simulink model "SkywalkerX8_AircraftModel_ROSGazeboAnimation"  (R2018a)
settings: Solver=FixedStepAuto  StartTime=0.0  StopTime=10  FixedStep=0.1  RelTol=1e-3
model workspace (MAT data in the model file):
  SL_ROS_VariableLengthArrays_MaxSizes.CommonInfo.ArrayTruncateAction = 'EmitWarning'
  SL_ROS_VariableLengthArrays_MaxSizes.MsgTypeMap = containers.Map
  SL_ROS_VariableLengthArrays_MaxSizes.MsgTypeMap.serialization.keys = {'gazebo_msgs/ModelState'}
  SL_ROS_VariableLengthArrays_MaxSizes.MsgTypeMap.serialization.values{1}(1).PropertyName = 'ModelName'
  SL_ROS_VariableLengthArrays_MaxSizes.MsgTypeMap.serialization.values{1}(1).DataType = 'uint8'
  SL_ROS_VariableLengthArrays_MaxSizes.MsgTypeMap.serialization.values{1}(1).MaxLength = 9
  SL_ROS_VariableLengthArrays_MaxSizes.MsgTypeMap.serialization.values{1}(2).PropertyName = 'ReferenceFrame'
  SL_ROS_VariableLengthArrays_MaxSizes.MsgTypeMap.serialization.values{1}(2).DataType = 'uint8'
  SL_ROS_VariableLengthArrays_MaxSizes.MsgTypeMap.serialization.values{1}(2).MaxLength = 128
  SL_ROS_VariableLengthArrays_MaxSizes.MsgTypeMap.serialization.uniformity = 0
  SL_ROS_VariableLengthArrays_MaxSizes.MsgTypeMap.serialization.keyType = 'char'
  SL_ROS_VariableLengthArrays_MaxSizes.MsgTypeMap.serialization.valueType = 'any'
undefined symbols (not defined in the file): ModelName, ModelName_SL_Info, Pose
libraries: robotlib x2, aerolibatmos2 x1, sharedtransform x1
settings Model: EnablePacing=on  Creator=David  LastModifiedBy=David

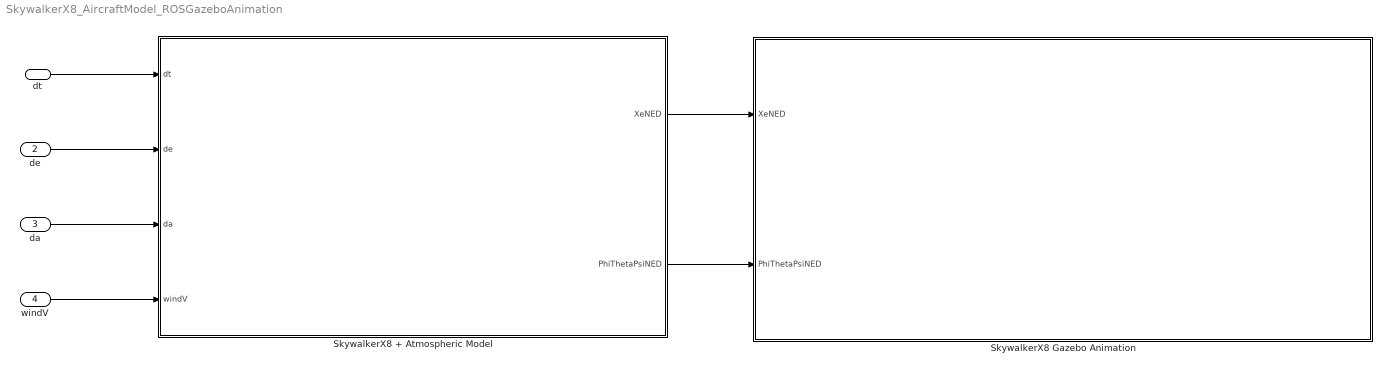
== system SkywalkerX8_AircraftModel_ROSGazeboAnimation ==
  dt : Inport
  de : Inport  Port=2
  da : Inport  Port=3
  windV : Inport  Port=4
  SkywalkerX8 + Atmospheric Model : Subsystem
      mask Display:
      | image('x8SkySunset.png', 'center')
      | 
      | port_label('input', 1, '\delta_t (Unitless)', 'texmode', 'on')
      | port_label('input', 2, '\delta_e (rad)', 'texmode', 'on')
      | port_label('input', 3, '\delta_a (rad)', 'texmode', 'on')
      | port_label('input', 4, '{\bf V_w^b} (m/s)', 'texmode', 'on')
      | 
      | port_label('output', 1, '{\bf X_e_{NED}} (m)', 'texmode', 'on')
      | port_label('output', 2, '(\phi \theta \psi)_{NED} (rad)', 'texmode', 'on')
  SkywalkerX8 Gazebo Animation : Subsystem
      mask Display:
      | image('skywalker_gazebo.png')
      | 
      | color('cyan')
      | 
      | port_label('input', 1, '{\bf X_e_{NED}} (m)', 'texmode', 'on')
      | port_label('input', 2, '(\phi \theta \psi)_{NED} (rad)', 'texmode', 'on')
  wires:
  dt/1 -> SkywalkerX8 + Atmospheric Model/1(dt)
  de/1 -> SkywalkerX8 + Atmospheric Model/2(de)
  da/1 -> SkywalkerX8 + Atmospheric Model/3(da)
  windV/1 -> SkywalkerX8 + Atmospheric Model/4(windV)
  SkywalkerX8 + Atmospheric Model/1(XeNED) -> SkywalkerX8 Gazebo Animation/1(XeNED)
  SkywalkerX8 + Atmospheric Model/2(PhiThetaPsiNED) -> SkywalkerX8 Gazebo Animation/2(PhiThetaPsiNED)

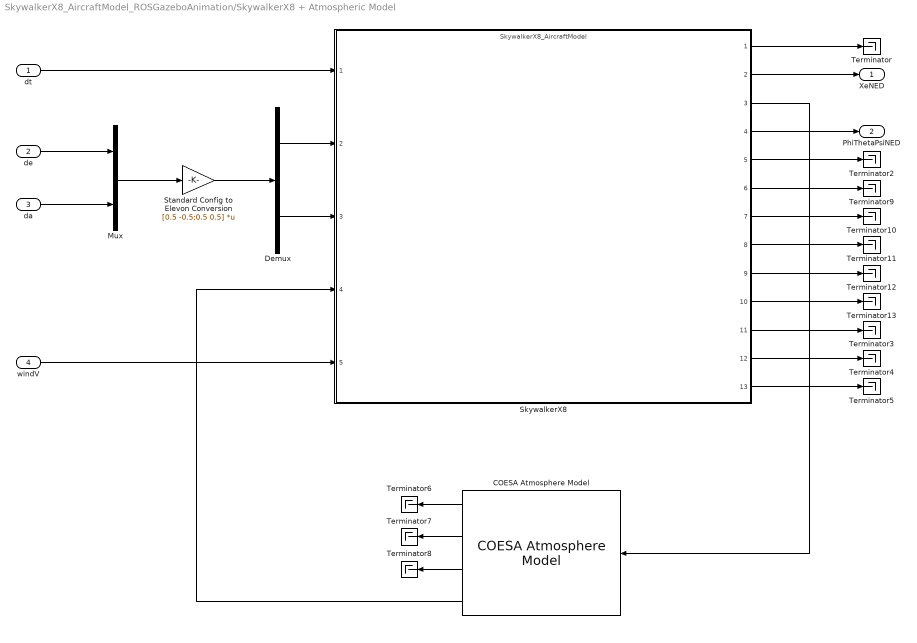
== system SkywalkerX8_AircraftModel_ROSGazeboAnimation/SkywalkerX8 + Atmospheric Model ==
  dt : Inport
  de : Inport  Port=2
  da : Inport  Port=3
  windV : Inport  Port=4
  COESA Atmosphere Model : aerolibatmos2/COESA Atmosphere Model  units=Metric (MKS)  spec=1976 COESA-extended U.S. Standard Atmosphere  model=Profile  profile_var=High temperature  profile_percent=1%  profile_alt=5 km (16404 ft)  envelope_var=High temperature  envelope_percent=1%  action=None
  Demux : Demux  Outputs=2
  Mux : Mux  Inputs=2
  SkywalkerX8 : ModelReference  ModelNameDialog=SkywalkerX8_AircraftModel  ModelReferenceVersion=1.162
      mask Display:
      | image('C:\MATLAB\masters\icons\Skywalker Main Block Icon.png', 'center')
      | 
      | color('cyan')
      | 
      | port_label('input', 1, 'k_{motor} (Unitless)', 'texmode', 'on')
      | port_label('input', 2, '\delta_{er} (rad)', 'texmode', 'on')
      | port_label('input', 3, '\delta_{el} (rad)', 'texmode', 'on')
      | port_label('input', 4, '\rho (kg/m^3)', 'texmode', 'on')
      | port_label('input', 5, '{\bf V_w^b} (m/s)', 'texmode', 'on')
      | 
      | port_label('output', 1, '{\bf V_e} (m/s)', 'texmode', 'on')
      | port_label('output', 2, '{\bf X_e} (m)', 'texmode', 'on')
      | port_label('output', 3, 'Altitude (m)', 'texmode', 'on')
      | port_label('output', 4, '\phi \theta \psi (rad)', 'texmode', 'on')
      | port_label('output', 5, 'R_{inertial}^{body}', 'texmode', 'on')
      | port_label('output', 6, 'V_a (m/s)', 'texmode', 'on')
      | port_label('output', 7, 'alpha (rad)', 'texmode', 'on')
      | port_label('output', 8, 'beta (rad)', 'texmode', 'on')
      | port_label('output', 9, '{\bf V_b} (m/s)', 'texmode', 'on')
      | port_label('output', 10, '{\bf \omega_b} (rad/s)', 'texmode', 'on')
      | port_label('output', 11, '{\bf \delta\omega_b/\deltat} (rad/s^2)', 'texmode', 'on')
      | port_label('output', 12, '{\bf a_{body}} (m/s^2)', 'texmode', 'on')
      | port_label('output', 13, '{\bf a_{inertial}} (m/s^2)', 'texmode', 'on')
  Standard Config to Elevon Conversion : Gain  Gain=[0.5 -0.5;0.5 0.5]  Multiplication=Matrix(K*u)
  Terminator{,2..13} (13 alike) : Terminator
  XeNED : Outport
  PhiThetaPsiNED : Outport  Port=2
  wires:
  SkywalkerX8/12 -> Terminator4/1
  COESA Atmosphere Model/2 -> Terminator7/1
  COESA Atmosphere Model/1 -> Terminator6/1
  Demux/2 -> SkywalkerX8/3
  SkywalkerX8/13 -> Terminator5/1
  COESA Atmosphere Model/3 -> Terminator8/1
  Mux/1 -> Standard Config to Elevon Conversion/1
  windV/1 -> SkywalkerX8/5
  SkywalkerX8/11 -> Terminator3/1
  SkywalkerX8/6 -> Terminator9/1
  COESA Atmosphere Model/4 -> SkywalkerX8/4
  SkywalkerX8/1 -> Terminator/1
  SkywalkerX8/5 -> Terminator2/1
  Standard Config to Elevon Conversion/1 -> Demux/1
  de/1 -> Mux/1
  Demux/1 -> SkywalkerX8/2
  SkywalkerX8/7 -> Terminator10/1
  dt/1 -> SkywalkerX8/1
  da/1 -> Mux/2
  SkywalkerX8/8 -> Terminator11/1
  SkywalkerX8/3 -> COESA Atmosphere Model/1
  SkywalkerX8/9 -> Terminator12/1
  SkywalkerX8/10 -> Terminator13/1
  SkywalkerX8/2 -> XeNED/1
  SkywalkerX8/4 -> PhiThetaPsiNED/1

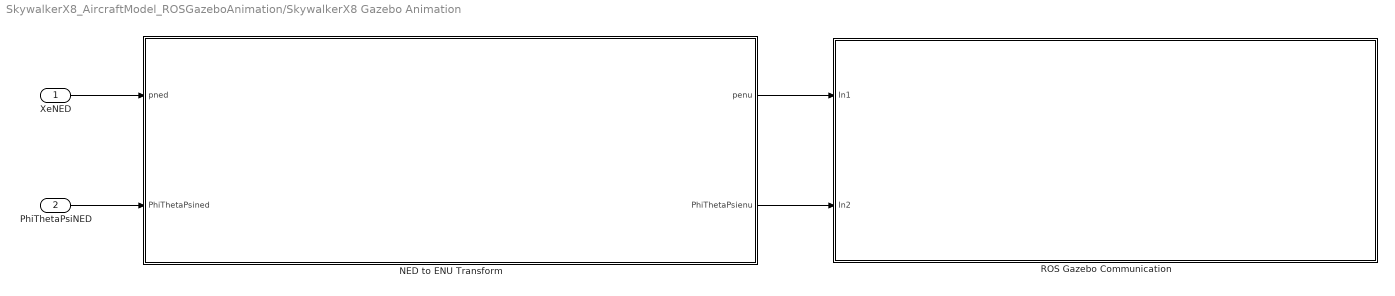
== system SkywalkerX8_AircraftModel_ROSGazeboAnimation/SkywalkerX8 Gazebo Animation ==
  XeNED : Inport
  PhiThetaPsiNED : Inport  Port=2
  "NED to ENU Transform " : Subsystem
      mask Display:
      | image('NEDtoENU.png', 'center')
      | 
      | port_label('input', 1, '{\bf X_e_{NED}} (m)', 'texmode', 'on')
      | port_label('input', 2, '(\phi \theta \psi)_{NED} (rad)', 'texmode', 'on')
      | 
      | port_label('output', 1, '{\bf X_e_{ENU}} (m)', 'texmode', 'on')
      | port_label('output', 2, '(\phi \theta \psi)_{ENU} (rad)', 'texmode', 'on')
  ROS Gazebo Communication : Subsystem
      mask Display:
      | image('rosToGazebo.png')
      | 
      | port_label('input', 1, '{\bf X_e_{ENU}} (m)', 'texmode', 'on')
      | port_label('input', 2, '(\phi \theta \psi)_{ENU} (rad)', 'texmode', 'on')
  wires:
  "NED to ENU Transform "/2(PhiThetaPsienu) -> ROS Gazebo Communication/2(In2)
  "NED to ENU Transform "/1(penu) -> ROS Gazebo Communication/1(In1)
  XeNED/1 -> "NED to ENU Transform "/1(pned)
  PhiThetaPsiNED/1 -> "NED to ENU Transform "/2(PhiThetaPsined)

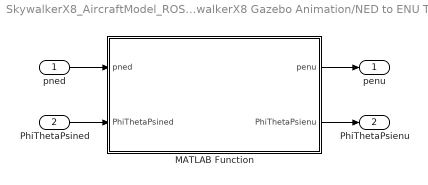
== system SkywalkerX8_AircraftModel_ROSGazeboAnimation/SkywalkerX8 Gazebo Animation/NED to ENU Transform  ==
  pned : Inport
  PhiThetaPsined : Inport  Port=2
  MATLAB Function : MATLAB Function  TreatAsAtomicUnit=on
  penu : Outport
  PhiThetaPsienu : Outport  Port=2
  wires:
  MATLAB Function/2(PhiThetaPsienu) -> PhiThetaPsienu/1
  pned/1 -> MATLAB Function/1(pned)
  MATLAB Function/1(penu) -> penu/1
  PhiThetaPsined/1 -> MATLAB Function/2(PhiThetaPsined)

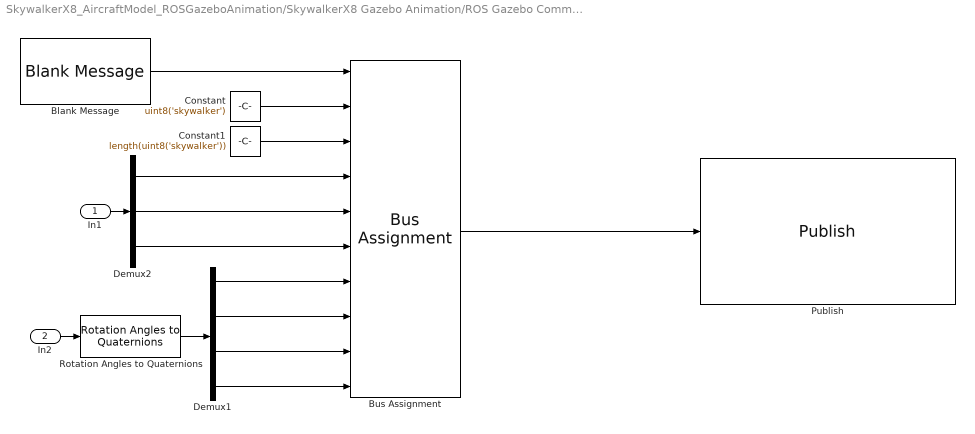
== system SkywalkerX8_AircraftModel_ROSGazeboAnimation/SkywalkerX8 Gazebo Animation/ROS Gazebo Communication ==
  In1 : Inport
  In2 : Inport  Port=2
  Blank Message : robotlib/Blank Message  SourceLibraryInfo=This block requires Robotics System Toolbox  messageType=gazebo_msgs/ModelState  SampleTime=inf
      settings: SourceProductBaseCode=RO
  Bus Assignment : BusAssignment  AssignedSignals=ModelName,ModelName_SL_Info.CurrentLength,Pose.Position.X,Pose.Position.Y,Pose.Position.Z,Pose.Orientation.W,Pose.Orientation.X,Pose.Orientation.Y,Pose.Orientation.Z
  Constant : Constant  Value=uint8('skywalker')
  Constant1 : Constant  Value=length(uint8('skywalker'))  OutDataTypeStr=uint32
  Demux1 : Demux
  Demux2 : Demux  Outputs=3
  Publish : robotlib/Publish  SourceLibraryInfo=This block requires Robotics System Toolbox  topicSource=Select from ROS network  topic=/gazebo/set_model_state  messageType=gazebo_msgs/ModelState  messageQueueLength=1
      settings: SourceProductBaseCode=RO
  Rotation Angles to Quaternions : sharedtransform/Rotation Angles to Quaternions  rotationOrder=XYZ  aMode=aMode
      settings: SourceProductName=Aerospace Blockset  SourceProductBaseCode=AE
  wires:
  Demux2/3 -> Bus Assignment/6
  Constant1/1 -> Bus Assignment/3
  Demux1/4 -> Bus Assignment/10
  Demux1/1 -> Bus Assignment/7
  In1/1 -> Demux2/1
  Demux2/1 -> Bus Assignment/4
  Demux1/2 -> Bus Assignment/8
  Bus Assignment/1 -> Publish/1
  In2/1 -> Rotation Angles to Quaternions/1
  Constant/1 -> Bus Assignment/2
  Blank Message/1 -> Bus Assignment/1
  Rotation Angles to Quaternions/1 -> Demux1/1
  Demux1/3 -> Bus Assignment/9
  Demux2/2 -> Bus Assignment/5

== matlab function SkywalkerX8_AircraftModel_ROSGazeboAnimation/SkywalkerX8 Gazebo Animation/NED to ENU Transform /MATLAB Function ==
  data: pned input size=[1, 3]; penu output size=[1, 3]; PhiThetaPsined input; PhiThetaPsienu output
function [penu, PhiThetaPsienu] = f_NEDtoENU(pned, PhiThetaPsined)

%% Description %%

% This function takes in global coordinates and rotation in the NED (North
% East Down) coordinate system, commonly used in aero applications, 
% and transforms this to the ENU (East North Up) coordinate system, commonly 
% used in robotics (and used by ROS for Gazebo simulations)

% This will be accomplished by swapping x and y, and inverting z and will
% be performed with a simple matrix transform of the form:

%                           Axned = xenu

% where A = [0 1 0
%            1 0 0
%            0 0 -1]

A = [0 1 0; 1 0 0; 0 0 -1]; % rotation matrix

penu = pned*A;
PhiThetaPsienu = PhiThetaPsined*A;

end
